simulink model "arduino_lab"  (R2017b)
settings: Solver=VariableStepAuto  StartTime=0.0  StopTime=500  RelTol=1e-3  EnableMultiTasking=on
StartFcn:
  | clear all
libraries: realtime_pacer_lib x1
settings Model: Creator=johnh  LastModifiedBy=johnh
settings OptimizationCC: LifeSpan=inf
settings DebuggingCC: SFUnexpectedBacktrackingDiag=warning  SFNoUnconditionalDefaultTransitionDiag=warning  SFExecutionAtInitializationDiag=none
settings CodeAppCC: StateflowObjectComments=on
settings GRTTargetCC: TargetLangStandard=C89/C90 (ANSI)  GeneratePreprocessorConditionals=Disable all
settings ConfigComp: CovMetricSettings=dw  CovHtmlReporting=on  CovSaveCumulativeToWorkspaceVar=on  CovSaveSingleToWorkspaceVar=on  CovExternalEMLEnable=off

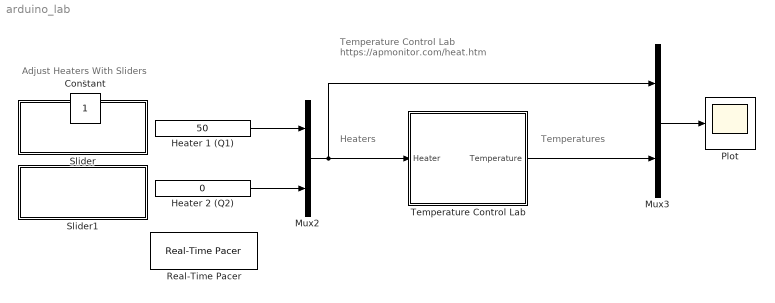
== system arduino_lab ==
  note: Adjust Heaters With Sliders
  note: Temperature Control Lab
      | https://apmonitor.com/heat.htm
  note: Heaters
  note: Temperatures
  Heater 1 (Q1) : Constant  Value=50
  Heater 2 (Q2) : Constant  Value=0
  Mux2 : Mux  Inputs=2
  Mux3 : Mux  Inputs=2
  Plot : Scope
  Real-Time Pacer : realtime_pacer_lib/Real-Time Pacer  simTimePerRealTime=1
  Slider : Subsystem  DialogController=hmiCreateDDGDialog  IsWebBlock=on  mask(MWDashboardBlock){webBlockId=e384a236-a50c-4b75-ba51-627058c2b810, webBlockType=slider, ShowInLibBrowser=on, ShowInitialText=on, HMISrcModelName=arduino_lab}
      mask prompts: webBlockId "WebBlock Id"; webBlockType "WebBlock Type"; HMISrcModelName "Source Model"
      mask help: SimulinkHMI:dialogs:SliderDialogDesc
      mask Help: helpview([docroot '/mapfiles/simulink.map'], 'hmi_slider')
      mask Display:
      | if strcmp(get_param(bdroot(gcb),'BlockDiagramType'), 'library')
      |     image([(matlabroot) '/toolbox/simulink/hmi/icons/Slider.png']);
      | end
  Slider1 : Subsystem  DialogController=hmiCreateDDGDialog  IsWebBlock=on  mask(MWDashboardBlock){webBlockId=e28f78d7-4053-462e-98b6-be5f9b67005a, webBlockType=slider, ShowInLibBrowser=on, ShowInitialText=on, HMISrcModelName=arduino_lab}
      mask prompts: webBlockId "WebBlock Id"; webBlockType "WebBlock Type"; HMISrcModelName "Source Model"
      mask help: SimulinkHMI:dialogs:SliderDialogDesc
      mask Help: helpview([docroot '/mapfiles/simulink.map'], 'hmi_slider')
      mask Display:
      | if strcmp(get_param(bdroot(gcb),'BlockDiagramType'), 'library')
      |     image([(matlabroot) '/toolbox/simulink/hmi/icons/Slider.png']);
      | end
  Temperature Control Lab : Subsystem
      mask Display: image('tclab.png');
  1 : Constant  IOType=siggen
  Constant : Constant  IOType=siggen
  wires:
  Heater 1 (Q1)/1 -> Mux2/1
  Heater 2 (Q2)/1 -> Mux2/2
  Temperature Control Lab/1(Temperature) -> Mux3/2
  Mux3/1 -> Plot/1
  Mux2/1 -> Mux3/1, Temperature Control Lab/1(Heater)

== system arduino_lab/Slider ==

== system arduino_lab/Slider1 ==

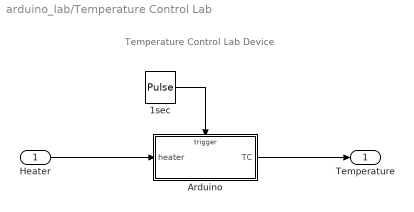
== system arduino_lab/Temperature Control Lab ==
  note: Temperature Control Lab Device
  Heater : Inport
  1sec : DiscretePulseGenerator  PulseType=Time based  Period=1  PulseWidth=50
  Arduino : Subsystem  TreatAsAtomicUnit=on
  Temperature : Outport
  wires:
  1sec/1 -> Arduino/Trigger
  Arduino/1(TC) -> Temperature/1
  Heater/1 -> Arduino/1(heater)

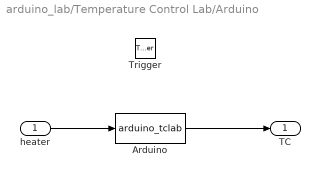
== system arduino_lab/Temperature Control Lab/Arduino ==
  heater : Inport  LatchByDelayingOutsideSignal=on
  Trigger : TriggerPort  VariantControl=Variant
  Arduino : MATLABFcn  MATLABFcn=arduino_tclab
  TC : Outport  InitialOutput=[23 23]
  wires:
  heater/1 -> Arduino/1
  Arduino/1 -> TC/1
